simulink model "NetworkModelIntermediateIntersectionSimpleDroneModel"  (R2018b)
settings: Solver=VariableStepAuto  StartTime=tStart  StopTime=tFinal  FixedStep=0.001  RelTol=1e-3
values from neighbouring files (symbols this model uses):
  bx = 50    [MotionModelling.m]
  by = 50    [MotionModelling.m]
  ConflictDrone1andDrone2 = ControlDetectionFunction(tout,PositionXDrone1TEST, PositionYDrone1TEST, PositionXDrone2TEST, PositionYDrone2TEST, ConflictDrone1andDrone2)    [ConflictDetectionTEST.m]
  ConflictDrone1andDrone3 = ControlDetectionFunction(tout,PositionXDrone1TEST, PositionYDrone1TEST, PositionXDrone3TEST, PositionYDrone3TEST, ConflictDrone1andDrone3)    [ConflictDetectionTEST.m]
  ConflictDrone1andDrone4 = ControlDetectionFunction(tout,PositionXDrone1TEST, PositionYDrone1TEST, PositionXDrone4TEST, PositionYDrone4TEST, ConflictDrone1andDrone4)    [ConflictDetectionTEST.m]
  ConflictDrone1andDrone5 = ControlDetectionFunction(tout,PositionXDrone1TEST, PositionYDrone1TEST, PositionXDrone5TEST, PositionYDrone5TEST, ConflictDrone1andDrone5)    [ConflictDetectionTEST.m]
  ConflictDrone1andDrone6 = ControlDetectionFunction(tout,PositionXDrone1TEST, PositionYDrone1TEST, PositionXDrone6TEST, PositionYDrone6TEST, ConflictDrone1andDrone6)    [ConflictDetectionTEST.m]
  ConflictDrone1andDrone7 = ControlDetectionFunction(tout,PositionXDrone1TEST, PositionYDrone1TEST, PositionXDrone7TEST, PositionYDrone7TEST, ConflictDrone1andDrone7)    [ConflictDetectionTEST.m]
  ConflictDrone2andDrone3 = ControlDetectionFunction(tout,PositionXDrone2TEST, PositionYDrone2TEST, PositionXDrone3TEST, PositionYDrone3TEST, ConflictDrone2andDrone3)    [ConflictDetectionTEST.m]
  ConflictDrone2andDrone4 = ControlDetectionFunction(tout,PositionXDrone2, PositionYDrone2, PositionXDrone4, PositionYDrone4, ConflictDrone2andDrone4)    [ConflictDetection.m]    (also in ConflictDetectionTEST.m = ControlDetectionFunction(tout,PositionXDrone2TEST, PositionY)
  ConflictDrone2andDrone5 = ControlDetectionFunction(tout,PositionXDrone2TEST, PositionYDrone2TEST, PositionXDrone5TEST, PositionYDrone5TEST, ConflictDrone2andDrone5)    [ConflictDetectionTEST.m]
  ConflictDrone2andDrone7 = ControlDetectionFunction(tout,PositionXDrone2TEST, PositionYDrone2TEST, PositionXDrone7TEST, PositionYDrone7TEST, ConflictDrone2andDrone7)    [ConflictDetectionTEST.m]
  ConflictDrone2andDrone8 = ControlDetectionFunction(tout,PositionXDrone2TEST, PositionYDrone2TEST, PositionXDrone8TEST, PositionYDrone8TEST, ConflictDrone2andDrone8)    [ConflictDetectionTEST.m]
  ConflictDrone3andDrone4 = ControlDetectionFunction(tout,PositionXDrone3TEST, PositionYDrone3TEST, PositionXDrone4TEST, PositionYDrone4TEST, ConflictDrone3andDrone4)    [ConflictDetectionTEST.m]
  ConflictDrone3andDrone5 = ControlDetectionFunction(tout,PositionXDrone3TEST, PositionYDrone3TEST, PositionXDrone5TEST, PositionYDrone5TEST, ConflictDrone3andDrone5)    [ConflictDetectionTEST.m]
  ConflictDrone3andDrone6 = ControlDetectionFunction(tout,PositionXDrone3TEST, PositionYDrone3TEST, PositionXDrone6TEST, PositionYDrone6TEST, ConflictDrone3andDrone6)    [ConflictDetectionTEST.m]
  ConflictDrone3andDrone7 = ControlDetectionFunction(tout,PositionXDrone3TEST, PositionYDrone3TEST, PositionXDrone7TEST, PositionYDrone7TEST, ConflictDrone3andDrone7)    [ConflictDetectionTEST.m]
  ConflictDrone4andDrone6 = ControlDetectionFunction(tout,PositionXDrone4TEST, PositionYDrone4TEST, PositionXDrone6TEST, PositionYDrone6TEST, ConflictDrone4andDrone6)    [ConflictDetectionTEST.m]
  ConflictDrone5andDrone7 = ControlDetectionFunction(tout,PositionXDrone5TEST, PositionYDrone5TEST, PositionXDrone7TEST, PositionYDrone7TEST, ConflictDrone5andDrone7)    [ConflictDetectionTEST.m]
  ConflictDrone5andDrone8 = ControlDetectionFunction(tout,PositionXDrone5TEST, PositionYDrone5TEST, PositionXDrone8TEST, PositionYDrone8TEST, ConflictDrone5andDrone8)    [ConflictDetectionTEST.m]
  ConflictDrone7andDrone8 = ControlDetectionFunction(tout,PositionXDrone7TEST, PositionYDrone7TEST, PositionXDrone8TEST, PositionYDrone8TEST, ConflictDrone7andDrone8)    [ConflictDetectionTEST.m]
  deltaVx1 = 0.1*cosd (theta2)    [MotionModelling.m]
  deltaVx2 = 0.12*cosd (theta2)    [MotionModelling.m]
  deltaVx3 = 0    [MotionModelling.m]
  deltaVx4 = -0.01*cosd (theta4)    [MotionModelling.m]
  deltaVx5 = 0.02*cosd (theta5)    [MotionModelling.m]
  deltaVx7 = 0    [MotionModelling.m]
  deltaVy1 = 0    [MotionModelling.m]
  deltaVy2 = 0.12*sind (theta2)    [MotionModelling.m]
  deltaVy3 = 0.03*sind (theta3)    [MotionModelling.m]
  deltaVy4 = -0.01*sind (theta4)    [MotionModelling.m]
  deltaVy5 = 0    [MotionModelling.m]
  deltaVy6 = -0.13*sind (theta6)    [MotionModelling.m]
  deltaVy7 = -0.04*sind (theta7)    [MotionModelling.m]
  m = 1.68    [DroneSubsystemModelling.m]    (also in MotionModelling.m = 1.38)
  VelocityStarX1 = vx10    [MotionModelling.m]
  VelocityStarX2 = vx20    [MotionModelling.m]
  VelocityStarX3 = vx30    [MotionModelling.m]
  VelocityStarX4 = vx40    [MotionModelling.m]
  VelocityStarX5 = vx50    [MotionModelling.m]
  VelocityStarX6 = vx60    [MotionModelling.m]
  VelocityStarX7 = vx70    [MotionModelling.m]
  VelocityStarX8 = vx80    [MotionModelling.m]
  VelocityStarY1 = vy10    [MotionModelling.m]
  VelocityStarY2 = vy20    [MotionModelling.m]
  VelocityStarY3 = vy30    [MotionModelling.m]
  VelocityStarY4 = vy40    [MotionModelling.m]
  VelocityStarY5 = vy50    [MotionModelling.m]
  VelocityStarY6 = vy60    [MotionModelling.m]
  VelocityStarY7 = vy70    [MotionModelling.m]
  VelocityStarY8 = vy80    [MotionModelling.m]
  vx10 = vin1*cosd (theta1)    [MotionModelling.m]
  vx20 = vin2*cosd (theta2)    [MotionModelling.m]
  vx30 = vin3*cosd (theta3)    [MotionModelling.m]
  vx40 = vin4*cosd (theta4)    [MotionModelling.m]
  vx50 = vin5*cosd (theta5)    [MotionModelling.m]
  vx60 = vin6*cosd (theta6)    [MotionModelling.m]
  vx70 = vin7*cosd (theta7)    [MotionModelling.m]
  vx80 = vin2*cosd (theta8)    [MotionModelling.m]
  vy10 = vin1*sind (theta1)    [MotionModelling.m]
  vy20 = vin2*sind (theta2)    [MotionModelling.m]
  vy30 = vin3*sind (theta3)    [MotionModelling.m]
  vy40 = vin4*sind (theta4)    [MotionModelling.m]
  vy50 = vin5*sind (theta5)    [MotionModelling.m]
  vy60 = vin6*sind (theta6)    [MotionModelling.m]
  vy70 = vin7*sind (theta7)    [MotionModelling.m]
  vy80 = vin2*sind (theta8)    [MotionModelling.m]
  x10 = 10    [MotionModelling.m]
  x20 = 10    [MotionModelling.m]
  x30 = 0    [MotionModelling.m]
  x40 = -10    [MotionModelling.m]
  x50 = -10    [MotionModelling.m]
  x60 = -10    [MotionModelling.m]
  x70 = 0    [MotionModelling.m]
  x80 = 10    [MotionModelling.m]
  y10 = 0    [MotionModelling.m]
  y20 = 10    [MotionModelling.m]
  y30 = 10    [MotionModelling.m]
  y40 = 10    [MotionModelling.m]
  y50 = 0    [MotionModelling.m]
  y60 = -10    [MotionModelling.m]
  y70 = -10    [MotionModelling.m]
  y80 = -10    [MotionModelling.m]
libraries: simulink x16
settings Model: Creator=CowUser  LastModifiedBy=n9544798

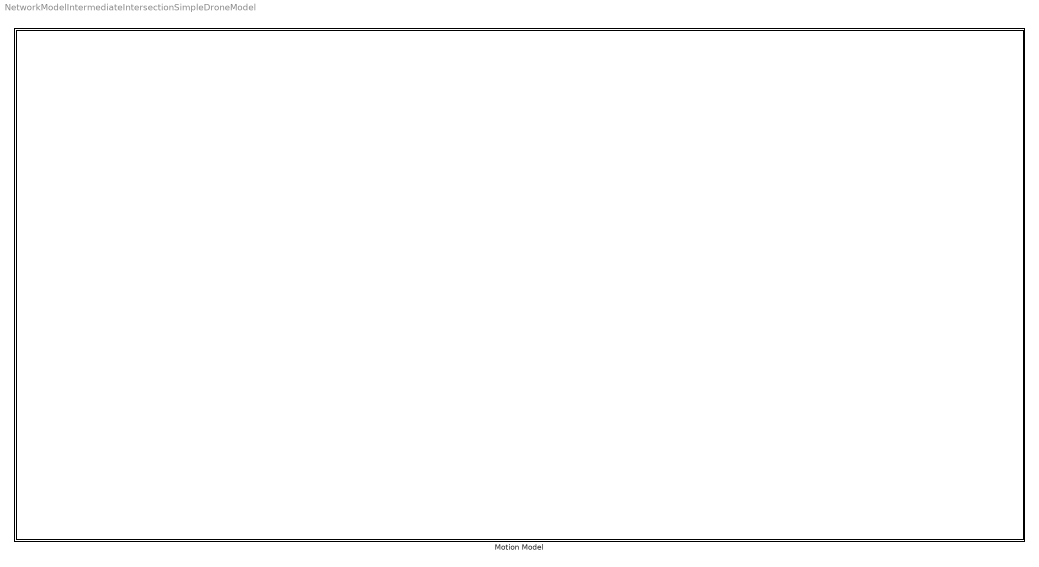
== system NetworkModelIntermediateIntersectionSimpleDroneModel ==
  Motion Model : Subsystem

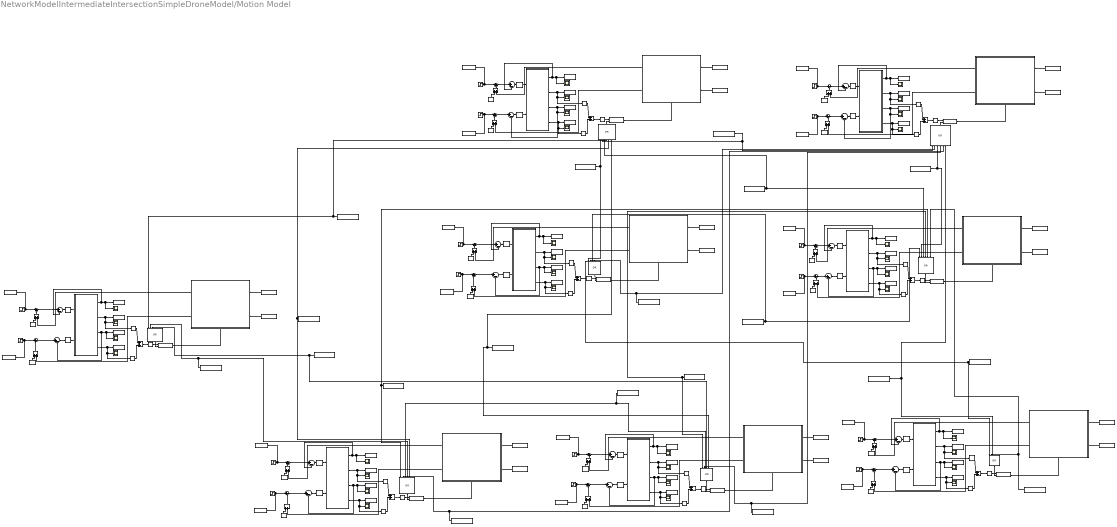
== system NetworkModelIntermediateIntersectionSimpleDroneModel/Motion Model ==
  note: Drone 2
  note: Intermediate Intersection
  note: Drone 4
  note: Sample 1
  note: Drone 1
  note: Drone 3
  note: Sample 2
  note: Sample 3
  note: Sample 4
  note: Sample 5
  note: Sample 6
  note: Sample 7
  note: Drone 5
  note: Sample 8
  note: Drone 7
  note: Sample 10
  note: Sample 9
  note: Sample 11
  note: Sample 13
  note: Sample 12
  note: Drone 6
  note: Sample 14
  note: Drone 4
  note: Sample 19
  note: Sample 18
  note: Sample 17
  note: Sample 16
  note: Sample 15
  Add{,1..23} (24 alike) : Sum
  Constant : Constant  Value=deltaVy2
  Constant1 : Constant  Value=ConflictDrone2andDrone4
  Constant10 : Constant  Value=ConflictDrone1andDrone3
  Constant11 : Constant  Value=deltaVy3
  Constant12 : Constant  Value=deltaVx1
  Constant{4..5,7..8,13..14,16..17,25..26,31..32,38..39,45..46} (16 alike) : Constant  Value=0
  Constant15 : Constant  Value=deltaVx3
  Constant18 : Constant  Value=ConflictDrone1andDrone4
  Constant19 : Constant  Value=ConflictDrone1andDrone2
  Constant2 : Constant  Value=deltaVy4
  Constant20 : Constant  Value=ConflictDrone3andDrone4
  Constant21 : Constant  Value=ConflictDrone2andDrone3
  Constant22 : Constant  Value=ConflictDrone1andDrone5
  Constant23 : Constant  Value=deltaVy5
  Constant24 : Constant  Value=deltaVx5
  Constant27 : Constant  Value=ConflictDrone3andDrone5
  Constant28 : Constant  Value=ConflictDrone1andDrone7
  Constant29 : Constant  Value=deltaVy7
  Constant3 : Constant  Value=deltaVx2
  Constant30 : Constant  Value=deltaVx7
  Constant33 : Constant  Value=ConflictDrone3andDrone7
  Constant34 : Constant  Value=ConflictDrone5andDrone7
  Constant35 : Constant  Value=ConflictDrone3andDrone6
  Constant36 : Constant  Value=deltaVy6
  Constant37 : Constant  Value=deltaVx5
  Constant40 : Constant  Value=ConflictDrone4andDrone6
  Constant41 : Constant  Value=ConflictDrone1andDrone6
  Constant42 : Constant  Value=ConflictDrone7andDrone8
  Constant43 : Constant  Value=deltaVy4
  Constant44 : Constant  Value=deltaVx4
  Constant47 : Constant  Value=ConflictDrone5andDrone8
  Constant48 : Constant  Value=ConflictDrone2andDrone8
  Constant49 : Constant  Value=ConflictDrone2andDrone7
  Constant50 : Constant  Value=ConflictDrone2andDrone5
  Constant6 : Constant  Value=deltaVx4
  Constant9 : Constant  Value=deltaVy1
  "Drone1 Subsystem " : Subsystem
  "Drone2 Subsystem " : Subsystem
  Drone3 Subsystem : Subsystem
  "Drone4 Subsystem " : Subsystem
  Drone5 Subsystem : Subsystem
  Drone6 Subsystem : Subsystem
  Drone7 Subsystem : Subsystem
  "Drone8 Subsystem " : Subsystem
  If Action Subsystem : Subsystem  TreatAsAtomicUnit=on
  If Action Subsystem1 : Subsystem  TreatAsAtomicUnit=on
  If Action Subsystem2 : Subsystem  TreatAsAtomicUnit=on
  If Action Subsystem3 : Subsystem  TreatAsAtomicUnit=on
  If Action Subsystem4 : Subsystem  TreatAsAtomicUnit=on
  If Action Subsystem5 : Subsystem  TreatAsAtomicUnit=on
  If Action Subsystem6 : Subsystem  TreatAsAtomicUnit=on
  If Action Subsystem7 : Subsystem  TreatAsAtomicUnit=on
  If{1..8} (8 alike) : If  NumInputs=2  IfExpression=(u1 <= R)&(u2 == 1)  ShowElse=off
  OR{,1..7} (8 alike) : Logic  Operator=OR  Inputs=7  IconShape=distinctive  AllPortsSameDT=off  OutDataTypeStr='double'
  PID Controller{1..16} (16 alike) : simulink/Continuous/PID Controller  Controller=PID  Form=Parallel  TimeDomain=Continuous-time  SampleTime=-1  IntegratorMethod=Forward Euler  FilterMethod=Forward Euler  ControllerParametersSource=internal  P=1.97139727738968e-05  I=1.5233344900537e-08  D=0.00566857635684116  UseFilter=on  N=15.1370363747334  TunerSelectOption=Transfer Function Based (PID Tuner App)  InitialConditionSource=internal  InitialConditionForIntegrator=0  InitialConditionForFilter=0  DifferentiatorICPrevScaledInput=0  ExternalReset=none  TrackingMode=off  Kt=1  LimitOutput=off  UpperSaturationLimit=inf  LowerSaturationLimit=-inf  LinearizeAsGain=on  AntiWindupMode=none  Kb=1  POutMin=[]  POutMax=[]  IOutMin=[]  IOutMax=[]  DOutMin=[]  DOutMax=[]  NOutMin=[]  NOutMax=[]  SumOutMin=[]  SumOutMax=[]  SaturationOutMin=[]  SaturationOutMax=[]  PParamMin=[]  PParamMax=[]  IParamMin=[]  IParamMax=[]  DParamMin=[]  DParamMax=[]  NParamMin=[]  NParamMax=[]  KbParamMin=[]  KbParamMax=[]  KtParamMin=[]  KtParamMax=[]  KbOutMin=[]  KbOutMax=[]  KtOutMin=[]  KtOutMax=[]  IntegratorOutMin=[]  IntegratorOutMax=[]  FilterOutMin=[]  FilterOutMax=[]  SumI1OutMin=[]  SumI1OutMax=[]  SumI2OutMin=[]  SumI2OutMax=[]  SumI3OutMin=[]  SumI3OutMax=[]  SumI4OutMin=[]  SumI4OutMax=[]  SumDOutMin=[]  SumDOutMax=[]  DifferentiatorOutMin=[]  DifferentiatorOutMax=[]  FilterDiffOutCoefMin=[]  FilterDiffOutCoefMax=[]  ReciprocalOutMin=[]  ReciprocalOutMax=[]  SumDenOutMin=[]  SumDenOutMax=[]  SumNumOutMin=[]  SumNumOutMax=[]  DivideOutMin=[]  DivideOutMax=[]  IntegratorContinuousStateAttributes=''  IntegratorStateMustResolveToSignalObject=off  IntegratorRTWStateStorageClass=Auto  FilterContinuousStateAttributes=''  FilterStateMustResolveToSignalObject=off  FilterRTWStateStorageClass=Auto  ParallelPVariant=InternalParameters  IdealPVariant=Disabled  IVariant=InternalParameters  DVariant=InternalParameters  IntegratorVariant=Continuous  SatVariant=Disabled  AWVariant=Passthrough  PCopyVariant=Disabled  TRVariant=Disabled  FdbkBlocksVariant=Forward  IdealPFdbkVariant=Disabled  SatFdbkVariant=Disabled  DerivativeFilterVariant=ContFilter  NVariant=InternalParameters  NCopyVariant=Disabled  FilterICVariant=InternalICsFilter  IntegratorICVariant=InternalICs  ExternalResetVariant=Disabled  TRSumVariant=Passthrough  SumFdbkVariant=Disabled  SumVariant=Sum_PID
  PositionXDrone{1..8} (8 alike) : Scope
  PositionYDrone{1..8} (8 alike) : Scope
  Sqrt{,1..7} (8 alike) : Sqrt  SaturateOnIntegerOverflow=on
  Square{,1..15} (16 alike) : Math  Operator=square  SaturateOnIntegerOverflow=on
  Step 1 : Step  Time=0  After=VelocityStarX2  SampleTime=0
  Step 10 : Step  Time=0  After=VelocityStarY5  SampleTime=0
  Step 11 : Step  Time=0  After=VelocityStarY7  SampleTime=0
  Step 12 : Step  Time=0  After=VelocityStarX7  SampleTime=0
  Step 13 : Step  Time=0  After=VelocityStarY6  SampleTime=0
  Step 14 : Step  Time=0  After=VelocityStarX6  SampleTime=0
  Step 15 : Step  Time=0  After=VelocityStarX8  SampleTime=0
  Step 16 : Step  Time=0  After=VelocityStarY8  SampleTime=0
  Step 2 : Step  Time=0  After=VelocityStarY2  SampleTime=0
  Step 3 : Step  Time=0  After=VelocityStarX1  SampleTime=0
  Step 4 : Step  Time=0  After=VelocityStarY1  SampleTime=0
  Step 5 : Step  Time=0  After=VelocityStarX3  SampleTime=0
  Step 6 : Step  Time=0  After=VelocityStarY3  SampleTime=0
  Step 7 : Step  Time=0  After=VelocityStarX4  SampleTime=0
  Step 8 : Step  Time=0  After=VelocityStarY4  SampleTime=0
  Step 9 : Step  Time=0  After=VelocityStarX5  SampleTime=0
  Sum{1..32} (32 alike) : Sum  Inputs=|+-
  To Workspace1 : ToWorkspace  VariableName=VelocityStarY2  SampleTime=-1
  To Workspace10 : ToWorkspace  VariableName=VelocityYDrone3  SampleTime=-1
  To Workspace11 : ToWorkspace  VariableName=PositionXDrone3  SampleTime=-1
  To Workspace12 : ToWorkspace  VariableName=VelocityXDrone3  SampleTime=-1
  To Workspace13 : ToWorkspace  VariableName=VelocityStarX3  SampleTime=-1
  To Workspace14 : ToWorkspace  VariableName=PositionYDrone3  SampleTime=-1
  To Workspace15 : ToWorkspace  VariableName=PositionXDrone1  SampleTime=-1
  To Workspace16 : ToWorkspace  VariableName=VelocityXDrone1  SampleTime=-1
  To Workspace17 : ToWorkspace  VariableName=VelocityStarX1  SampleTime=-1
  To Workspace18 : ToWorkspace  VariableName=PositionYDrone1  SampleTime=-1
  To Workspace19 : ToWorkspace  VariableName=VelocityStarY4  SampleTime=-1
  To Workspace2 : ToWorkspace  VariableName=VelocityYDrone2  SampleTime=-1
  To Workspace20 : ToWorkspace  VariableName=VelocityYDrone4  SampleTime=-1
  To Workspace21 : ToWorkspace  VariableName=PositionXDrone4  SampleTime=-1
  To Workspace22 : ToWorkspace  VariableName=VelocityXDrone4  SampleTime=-1
  To Workspace23 : ToWorkspace  VariableName=VelocityStarX4  SampleTime=-1
  To Workspace24 : ToWorkspace  VariableName=PositionYDrone4  SampleTime=-1
  To Workspace25 : ToWorkspace  VariableName=VelocityStarY5  SampleTime=-1
  To Workspace26 : ToWorkspace  VariableName=VelocityYDrone5  SampleTime=-1
  To Workspace27 : ToWorkspace  VariableName=PositionXDrone5  SampleTime=-1
  To Workspace28 : ToWorkspace  VariableName=VelocityXDrone5  SampleTime=-1
  To Workspace29 : ToWorkspace  VariableName=VelocityStarX5  SampleTime=-1
  To Workspace3 : ToWorkspace  VariableName=PositionXDrone2  SampleTime=-1
  To Workspace30 : ToWorkspace  VariableName=PositionYDrone5  SampleTime=-1
  To Workspace31 : ToWorkspace  VariableName=VelocityStarY7  SampleTime=-1
  To Workspace32 : ToWorkspace  VariableName=VelocityYDrone7  SampleTime=-1
  To Workspace33 : ToWorkspace  VariableName=PositionXDrone7  SampleTime=-1
  To Workspace34 : ToWorkspace  VariableName=VelocityXDrone7  SampleTime=-1
  To Workspace35 : ToWorkspace  VariableName=VelocityStarX7  SampleTime=-1
  To Workspace36 : ToWorkspace  VariableName=PositionYDrone7  SampleTime=-1
  To Workspace37 : ToWorkspace  VariableName=VelocityStarY6  SampleTime=-1
  To Workspace38 : ToWorkspace  VariableName=VelocityYDrone6  SampleTime=-1
  To Workspace39 : ToWorkspace  VariableName=PositionXDrone6  SampleTime=-1
  To Workspace4 : ToWorkspace  VariableName=VelocityXDrone2  SampleTime=-1
  To Workspace40 : ToWorkspace  VariableName=VelocityXDrone6  SampleTime=-1
  To Workspace41 : ToWorkspace  VariableName=VelocityStarX6  SampleTime=-1
  To Workspace42 : ToWorkspace  VariableName=PositionYDrone6  SampleTime=-1
  To Workspace43 : ToWorkspace  VariableName=VelocityStarY8  SampleTime=-1
  To Workspace44 : ToWorkspace  VariableName=VelocityYDrone8  SampleTime=-1
  To Workspace45 : ToWorkspace  VariableName=PositionXDrone8  SampleTime=-1
  To Workspace46 : ToWorkspace  VariableName=VelocityXDrone8  SampleTime=-1
  To Workspace47 : ToWorkspace  VariableName=VelocityStarX8  SampleTime=-1
  To Workspace48 : ToWorkspace  VariableName=PositionYDrone8  SampleTime=-1
  To Workspace5 : ToWorkspace  VariableName=VelocityStarX2  SampleTime=-1
  To Workspace6 : ToWorkspace  VariableName=PositionYDrone2  SampleTime=-1
  To Workspace7 : ToWorkspace  VariableName=VelocityStarY1  SampleTime=-1
  To Workspace8 : ToWorkspace  VariableName=VelocityStarY3  SampleTime=-1
  To Workspace9 : ToWorkspace  VariableName=VelocityYDrone1  SampleTime=-1
  VelocityXDrone{1..8} (8 alike) : Scope
  VelocityYDrone{1..8} (8 alike) : Scope
  wires:
  "Drone2 Subsystem "/3(VelocityY) -> Sum1/2, VelocityYDrone2/1, To Workspace2/1
  Sum1/1 -> PID Controller1/1
  PID Controller7/1 -> "Drone2 Subsystem "/1(InputForceX)
  "Drone2 Subsystem "/4(PositionY) -> Square1/1, PositionYDrone2/1, To Workspace6/1
  "Drone2 Subsystem "/2(PositionX) -> Square/1, PositionXDrone2/1, To Workspace3/1
  PID Controller1/1 -> "Drone2 Subsystem "/2(InputForceY)
  "Drone2 Subsystem "/1(VelocityX) -> VelocityXDrone2/1, To Workspace4/1, Sum2/2
  Step 7/1 -> Sum6/1, To Workspace23/1
  Step 8/1 -> To Workspace19/1, Sum7/1
  Square/1 -> Add/1
  Square1/1 -> Add/2
  Add/1 -> Sqrt/1
  Sqrt/1 -> If3/1
  Square2/1 -> Add1/1
  Add1/1 -> Sqrt1/1
  "Drone4 Subsystem "/2(PositionX) -> Square2/1, PositionXDrone4/1, To Workspace21/1
  Square3/1 -> Add1/2
  "Drone4 Subsystem "/4(PositionY) -> Square3/1, PositionYDrone4/1, To Workspace24/1
  Sqrt1/1 -> If1/1
  Sum2/1 -> PID Controller7/1
  Constant/1 -> If Action Subsystem/2(deltaVy2)
  Constant3/1 -> If Action Subsystem/1(deltaVx2)
  Step 1/1 -> Sum9/1, To Workspace5/1
  Sum10/1 -> Sum1/1
  Step 2/1 -> Sum10/1, To Workspace1/1
  If Action Subsystem/1(dVx2) -> Add3/2
  If Action Subsystem/2(dVy2) -> Add2/2
  If3/1 -> If Action Subsystem/Action
  Constant4/1 -> Add3/1
  Constant5/1 -> Add2/1
  Add2/1 -> Sum10/2
  Constant1/1 -> OR1/1, OR2/1
  If1/1 -> If Action Subsystem1/Action
  If Action Subsystem1/1(dVx4) -> Add4/2
  Constant2/1 -> If Action Subsystem1/2(deltaVy4)
  Constant6/1 -> If Action Subsystem1/1(deltaVx4)
  Add4/1 -> Sum6/2
  Constant7/1 -> Add4/1
  Sum3/1 -> PID Controller6/1
  "Drone4 Subsystem "/1(VelocityX) -> Sum3/2, To Workspace22/1, VelocityXDrone4/1
  Constant8/1 -> Add5/1
  If Action Subsystem1/2(dVy4) -> Add5/2
  "Drone4 Subsystem "/3(VelocityY) -> Sum4/2, VelocityYDrone4/1, To Workspace20/1
  Sum4/1 -> PID Controller3/1
  Add3/1 -> Sum9/2
  Sum9/1 -> Sum2/1
  Step 3/1 -> Sum16/1, To Workspace17/1
  Add9/1 -> Sum16/2
  "Drone1 Subsystem "/4(PositionY) -> Square5/1, PositionYDrone1/1, To Workspace18/1
  Drone3 Subsystem/3(VelocityY) -> Sum13/2, VelocityYDrone3/1, To Workspace10/1
  Constant17/1 -> Add11/1
  Add10/1 -> Sum14/2
  Sum15/1 -> Sum13/1
  If Action Subsystem3/2(dVy3) -> Add11/2
  Add11/1 -> Sum15/2
  Sum11/1 -> PID Controller8/1
  Constant10/1 -> OR3/2, OR/3
  If Action Subsystem2/1(dVx1) -> Add9/2
  Constant11/1 -> If Action Subsystem3/2(deltaVy3)
  Constant13/1 -> Add9/1
  Sqrt3/1 -> If2/1
  Constant16/1 -> Add10/1
  Add8/1 -> Sum8/2
  Drone3 Subsystem/1(VelocityX) -> Sum12/2, To Workspace12/1, VelocityXDrone3/1
  Constant14/1 -> Add8/1
  If2/1 -> If Action Subsystem3/Action
  If Action Subsystem3/1(dVx3) -> Add10/2
  Drone3 Subsystem/4(PositionY) -> Square7/1, PositionYDrone3/1, To Workspace14/1
  Constant12/1 -> If Action Subsystem2/1(deltaVx1)
  Constant15/1 -> If Action Subsystem3/1(deltaVx3)
  Step 4/1 -> Sum8/1, To Workspace7/1
  "Drone1 Subsystem "/2(PositionX) -> Square4/1, PositionXDrone1/1, To Workspace15/1
  Add7/1 -> Sqrt3/1
  Square6/1 -> Add7/1
  Square5/1 -> Add6/2
  Constant9/1 -> If Action Subsystem2/2(deltaVy1)
  Square7/1 -> Add7/2
  Sum13/1 -> PID Controller5/1
  Drone3 Subsystem/2(PositionX) -> Square6/1, PositionXDrone3/1, To Workspace11/1
  Sum14/1 -> Sum12/1
  Step 5/1 -> Sum14/1, To Workspace13/1
  Sum12/1 -> PID Controller4/1
  Step 6/1 -> To Workspace8/1, Sum15/1
  Sum5/1 -> PID Controller2/1
  Sqrt2/1 -> If4/1
  PID Controller4/1 -> Drone3 Subsystem/1(InputForceX)
  Add6/1 -> Sqrt2/1
  PID Controller5/1 -> Drone3 Subsystem/2(InputForceY)
  "Drone1 Subsystem "/3(VelocityY) -> Sum5/2, VelocityYDrone1/1, To Workspace9/1
  If Action Subsystem2/2(dVy1) -> Add8/2
  Square4/1 -> Add6/1
  If4/1 -> If Action Subsystem2/Action
  "Drone1 Subsystem "/1(VelocityX) -> VelocityXDrone1/1, To Workspace16/1, Sum11/2
  OR/1 -> If4/2
  Constant18/1 -> OR/2, OR1/2
  OR1/1 -> If1/2
  OR2/1 -> If3/2
  Constant19/1 -> OR2/2, OR/1
  Constant20/1 -> OR3/1, OR1/3
  OR3/1 -> If2/2
  Constant21/1 -> OR3/3, OR2/3
  Sum6/1 -> Sum3/1
  Sum8/1 -> Sum5/1
  Sum16/1 -> Sum11/1
  Add5/1 -> Sum7/2
  Sum7/1 -> Sum4/1
  PID Controller6/1 -> "Drone4 Subsystem "/1(InputForceX)
  PID Controller3/1 -> "Drone4 Subsystem "/2(InputForceY)
  Constant26/1 -> Add14/1
  Constant25/1 -> Add13/1
  Sum17/1 -> PID Controller10/1
  Drone5 Subsystem/1(VelocityX) -> Sum17/2, To Workspace28/1, VelocityXDrone5/1
  Drone5 Subsystem/2(PositionX) -> Square8/1, PositionXDrone5/1, To Workspace27/1
  Step 10/1 -> To Workspace25/1, Sum20/1
  Square8/1 -> Add12/1
  PID Controller10/1 -> Drone5 Subsystem/1(InputForceX)
  Drone5 Subsystem/3(VelocityY) -> Sum18/2, VelocityYDrone5/1, To Workspace26/1
  Sum20/1 -> Sum18/1
  Sqrt4/1 -> If5/1
  If5/1 -> If Action Subsystem4/Action
  Sum18/1 -> PID Controller9/1
  PID Controller9/1 -> Drone5 Subsystem/2(InputForceY)
  Sum19/1 -> Sum17/1
  If Action Subsystem4/1(dVx5) -> Add13/2
  Add14/1 -> Sum20/2
  Constant23/1 -> If Action Subsystem4/2(deltaVy5)
  Constant22/1 -> OR/4, OR4/2
  Step 9/1 -> Sum19/1, To Workspace29/1
  If Action Subsystem4/2(dVy5) -> Add14/2
  Square9/1 -> Add12/2
  Constant24/1 -> If Action Subsystem4/1(deltaVx5)
  Drone5 Subsystem/4(PositionY) -> Square9/1, PositionYDrone5/1, To Workspace30/1
  Add13/1 -> Sum19/2
  OR4/1 -> If5/2
  Add12/1 -> Sqrt4/1
  Constant27/1 -> OR3/4, OR4/1
  OR5/1 -> If6/2
  Constant30/1 -> If Action Subsystem5/1(deltaVx7)
  Drone7 Subsystem/4(PositionY) -> Square11/1, PositionYDrone7/1, To Workspace36/1
  If Action Subsystem5/2(dVy7) -> Add17/2
  Add16/1 -> Sum23/2
  Add15/1 -> Sqrt5/1
  Constant28/1 -> OR/5, OR5/2
  Constant29/1 -> If Action Subsystem5/2(deltaVy7)
  Square11/1 -> Add15/2
  Add17/1 -> Sum24/2
  If Action Subsystem5/1(dVx7) -> Add16/2
  Constant34/1 -> OR4/3, OR5/3
  Constant33/1 -> OR3/5, OR5/1
  Sum22/1 -> PID Controller12/1
  Sum24/1 -> Sum22/1
  If6/1 -> If Action Subsystem5/Action
  Step 12/1 -> Sum23/1, To Workspace35/1
  Drone7 Subsystem/3(VelocityY) -> Sum22/2, VelocityYDrone7/1, To Workspace32/1
  Drone7 Subsystem/2(PositionX) -> Square10/1, PositionXDrone7/1, To Workspace33/1
  PID Controller11/1 -> Drone7 Subsystem/1(InputForceX)
  Square10/1 -> Add15/1
  Step 11/1 -> To Workspace31/1, Sum24/1
  Constant31/1 -> Add16/1
  Sum21/1 -> PID Controller11/1
  Sqrt5/1 -> If6/1
  Drone7 Subsystem/1(VelocityX) -> Sum21/2, To Workspace34/1, VelocityXDrone7/1
  Sum23/1 -> Sum21/1
  Constant32/1 -> Add17/1
  Add20/1 -> Sum28/2
  Square12/1 -> Add18/1
  Sum27/1 -> Sum25/1
  PID Controller14/1 -> Drone6 Subsystem/2(InputForceY)
  Square13/1 -> Add18/2
  PID Controller13/1 -> Drone6 Subsystem/1(InputForceX)
  Drone6 Subsystem/3(VelocityY) -> Sum26/2, VelocityYDrone6/1, To Workspace38/1
  Drone6 Subsystem/4(PositionY) -> Square13/1, PositionYDrone6/1, To Workspace42/1
  Constant38/1 -> Add19/1
  Constant40/1 -> OR1/4, OR6/1
  OR6/1 -> If7/2
  Sum25/1 -> PID Controller13/1
  Sqrt6/1 -> If7/1
  If Action Subsystem6/2(dVy6) -> Add20/2
  Constant35/1 -> OR3/6, OR6/2
  Constant39/1 -> Add20/1
  Sum28/1 -> Sum26/1
  If Action Subsystem6/1(dVx6) -> Add19/2
  Step 13/1 -> To Workspace37/1, Sum28/1
  If7/1 -> If Action Subsystem6/Action
  Constant41/1 -> OR6/3, OR/6
  Add19/1 -> Sum27/2
  Step 14/1 -> Sum27/1, To Workspace41/1
  Sum26/1 -> PID Controller14/1
  Drone6 Subsystem/2(PositionX) -> Square12/1, PositionXDrone6/1, To Workspace39/1
  Add18/1 -> Sqrt6/1
  Constant36/1 -> If Action Subsystem6/2(deltaVy6)
  Constant37/1 -> If Action Subsystem6/1(deltaVx6)
  Drone6 Subsystem/1(VelocityX) -> Sum25/2, To Workspace40/1, VelocityXDrone6/1
  Step 16/1 -> To Workspace43/1, Sum32/1
  If Action Subsystem7/1(dVx4) -> Add22/2
  Constant48/1 -> OR2/4, OR7/1
  Constant43/1 -> If Action Subsystem7/2(deltaVy4)
  Add21/1 -> Sqrt7/1
  Square14/1 -> Add21/1
  Constant46/1 -> Add23/1
  If8/1 -> If Action Subsystem7/Action
  Sum30/1 -> PID Controller15/1
  "Drone8 Subsystem "/1(VelocityX) -> Sum29/2, To Workspace46/1, VelocityXDrone8/1
  Constant47/1 -> OR4/4, OR7/3
  "Drone8 Subsystem "/3(VelocityY) -> Sum30/2, VelocityYDrone8/1, To Workspace44/1
  "Drone8 Subsystem "/2(PositionX) -> Square14/1, PositionXDrone8/1, To Workspace45/1
  Sqrt7/1 -> If8/1
  Add23/1 -> Sum32/2
  OR7/1 -> If8/2
  PID Controller15/1 -> "Drone8 Subsystem "/2(InputForceY)
  If Action Subsystem7/2(dVy4) -> Add23/2
  Square15/1 -> Add21/2
  Sum32/1 -> Sum30/1
  Constant45/1 -> Add22/1
  "Drone8 Subsystem "/4(PositionY) -> Square15/1, PositionYDrone8/1, To Workspace48/1
  Constant44/1 -> If Action Subsystem7/1(deltaVx4)
  Step 15/1 -> Sum31/1, To Workspace47/1
  Sum29/1 -> PID Controller16/1
  Add22/1 -> Sum31/2
  PID Controller16/1 -> "Drone8 Subsystem "/1(InputForceX)
  Sum31/1 -> Sum29/1
  Constant42/1 -> OR5/4, OR7/2
  Constant49/1 -> OR2/5, OR5/5
  Constant50/1 -> OR2/6, OR4/5
  PID Controller8/1 -> "Drone1 Subsystem "/1(InputForceX)
  PID Controller2/1 -> "Drone1 Subsystem "/2(InputForceY)
  PID Controller12/1 -> Drone7 Subsystem/2(InputForceY)

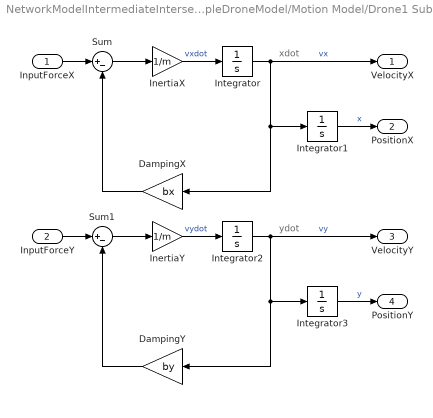
== system NetworkModelIntermediateIntersectionSimpleDroneModel/Motion Model/Drone1 Subsystem  ==
  note: ydot
  note: xdot
  InputForceX : Inport
  InputForceY : Inport  Port=2
  DampingX : Gain  Gain=bx
  DampingY : Gain  Gain=by
  InertiaX : Gain  Gain=1/m
  InertiaY : Gain  Gain=1/m
  Integrator : Integrator  InitialCondition=vx10
  Integrator1 : Integrator  InitialCondition=x10
  Integrator2 : Integrator  InitialCondition=vy10
  Integrator3 : Integrator  InitialCondition=y10
  Sum : Sum  Inputs=|+-
  Sum1 : Sum  Inputs=|+-
  VelocityX : Outport
  PositionX : Outport  Port=2
  VelocityY : Outport  Port=3
  PositionY : Outport  Port=4
  wires:
  InertiaX/1 -> Integrator/1  "vxdot"
  Integrator1/1 -> PositionX/1  "x"
  InputForceY/1 -> Sum1/1
  Integrator2/1 -> VelocityY/1, Integrator3/1, DampingY/1  "vy"
  InertiaY/1 -> Integrator2/1  "vydot"
  Integrator/1 -> VelocityX/1, Integrator1/1, DampingX/1  "vx"
  Sum1/1 -> InertiaY/1
  DampingY/1 -> Sum1/2
  Sum/1 -> InertiaX/1
  DampingX/1 -> Sum/2
  Integrator3/1 -> PositionY/1  "y"
  InputForceX/1 -> Sum/1

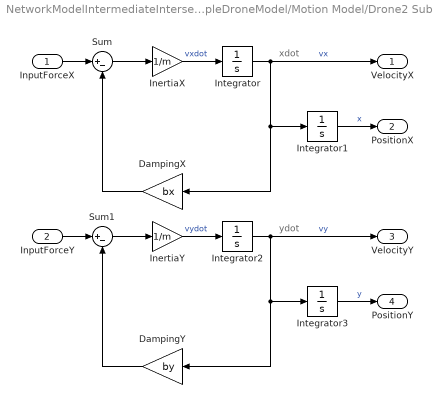
== system NetworkModelIntermediateIntersectionSimpleDroneModel/Motion Model/Drone2 Subsystem  ==
  note: ydot
  note: xdot
  InputForceX : Inport
  InputForceY : Inport  Port=2
  "DampingX " : Gain  Gain=bx
  DampingY : Gain  Gain=by
  InertiaX : Gain  Gain=1/m
  InertiaY : Gain  Gain=1/m
  Integrator : Integrator  InitialCondition=vx20
  Integrator1 : Integrator  InitialCondition=x20
  Integrator2 : Integrator  InitialCondition=vy20
  Integrator3 : Integrator  InitialCondition=y20
  Sum : Sum  Inputs=|+-
  Sum1 : Sum  Inputs=|+-
  VelocityX : Outport
  PositionX : Outport  Port=2
  VelocityY : Outport  Port=3
  PositionY : Outport  Port=4
  wires:
  InputForceY/1 -> Sum1/1
  Integrator2/1 -> VelocityY/1, Integrator3/1, DampingY/1  "vy"
  DampingY/1 -> Sum1/2
  InertiaY/1 -> Integrator2/1  "vydot"
  Integrator1/1 -> PositionX/1  "x"
  Integrator/1 -> VelocityX/1, Integrator1/1, "DampingX "/1  "vx"
  InputForceX/1 -> Sum/1
  Sum/1 -> InertiaX/1
  Integrator3/1 -> PositionY/1  "y"
  "DampingX "/1 -> Sum/2
  InertiaX/1 -> Integrator/1  "vxdot"
  Sum1/1 -> InertiaY/1

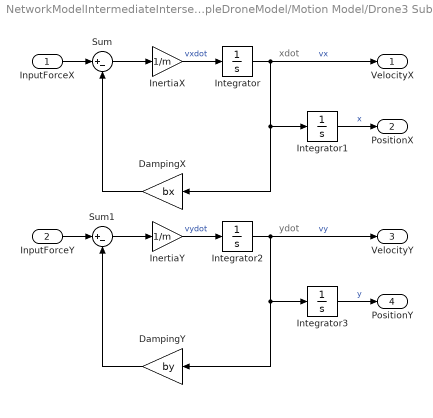
== system NetworkModelIntermediateIntersectionSimpleDroneModel/Motion Model/Drone3 Subsystem ==
  note: xdot
  note: ydot
  InputForceX : Inport
  InputForceY : Inport  Port=2
  DampingX : Gain  Gain=bx
  DampingY : Gain  Gain=by
  InertiaX : Gain  Gain=1/m
  InertiaY : Gain  Gain=1/m
  Integrator : Integrator  InitialCondition=vx30
  Integrator1 : Integrator  InitialCondition=x30
  Integrator2 : Integrator  InitialCondition=vy30
  Integrator3 : Integrator  InitialCondition=y30
  Sum : Sum  Inputs=|+-
  Sum1 : Sum  Inputs=|+-
  VelocityX : Outport
  PositionX : Outport  Port=2
  VelocityY : Outport  Port=3
  PositionY : Outport  Port=4
  wires:
  Integrator3/1 -> PositionY/1  "y"
  Integrator/1 -> VelocityX/1, Integrator1/1, DampingX/1  "vx"
  InertiaY/1 -> Integrator2/1  "vydot"
  DampingY/1 -> Sum1/2
  Sum1/1 -> InertiaY/1
  Integrator1/1 -> PositionX/1  "x"
  InputForceY/1 -> Sum1/1
  DampingX/1 -> Sum/2
  Sum/1 -> InertiaX/1
  InertiaX/1 -> Integrator/1  "vxdot"
  InputForceX/1 -> Sum/1
  Integrator2/1 -> VelocityY/1, Integrator3/1, DampingY/1  "vy"

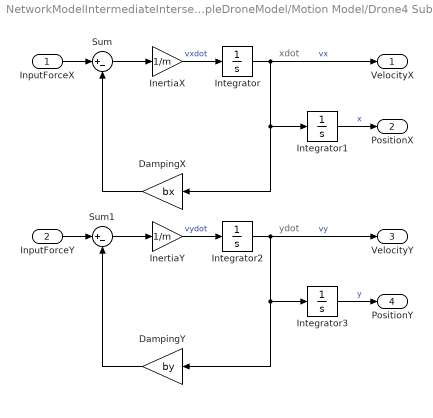
== system NetworkModelIntermediateIntersectionSimpleDroneModel/Motion Model/Drone4 Subsystem  ==
  note: xdot
  note: ydot
  InputForceX : Inport
  InputForceY : Inport  Port=2
  "DampingX " : Gain  Gain=bx
  DampingY : Gain  Gain=by
  InertiaX : Gain  Gain=1/m
  InertiaY : Gain  Gain=1/m
  Integrator : Integrator  InitialCondition=vx40
  Integrator1 : Integrator  InitialCondition=x40
  Integrator2 : Integrator  InitialCondition=vy40
  Integrator3 : Integrator  InitialCondition=y40
  Sum : Sum  Inputs=|+-
  Sum1 : Sum  Inputs=|+-
  VelocityX : Outport
  PositionX : Outport  Port=2
  VelocityY : Outport  Port=3
  PositionY : Outport  Port=4
  wires:
  Integrator1/1 -> PositionX/1  "x"
  InputForceX/1 -> Sum/1
  InertiaY/1 -> Integrator2/1  "vydot"
  InputForceY/1 -> Sum1/1
  Integrator3/1 -> PositionY/1  "y"
  Integrator2/1 -> VelocityY/1, Integrator3/1, DampingY/1  "vy"
  "DampingX "/1 -> Sum/2
  InertiaX/1 -> Integrator/1  "vxdot"
  Sum1/1 -> InertiaY/1
  Sum/1 -> InertiaX/1
  Integrator/1 -> VelocityX/1, Integrator1/1, "DampingX "/1  "vx"
  DampingY/1 -> Sum1/2

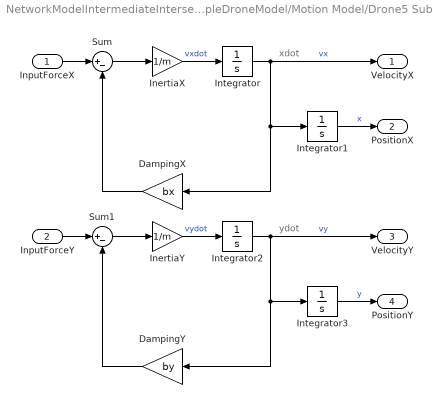
== system NetworkModelIntermediateIntersectionSimpleDroneModel/Motion Model/Drone5 Subsystem ==
  note: xdot
  note: ydot
  InputForceX : Inport
  InputForceY : Inport  Port=2
  "DampingX " : Gain  Gain=bx
  DampingY : Gain  Gain=by
  InertiaX : Gain  Gain=1/m
  InertiaY : Gain  Gain=1/m
  Integrator : Integrator  InitialCondition=vx50
  Integrator1 : Integrator  InitialCondition=x50
  Integrator2 : Integrator  InitialCondition=vy50
  Integrator3 : Integrator  InitialCondition=y50
  Sum : Sum  Inputs=|+-
  Sum1 : Sum  Inputs=|+-
  VelocityX : Outport
  PositionX : Outport  Port=2
  VelocityY : Outport  Port=3
  PositionY : Outport  Port=4
  wires:
  Integrator/1 -> VelocityX/1, Integrator1/1, "DampingX "/1  "vx"
  Sum/1 -> InertiaX/1
  Sum1/1 -> InertiaY/1
  "DampingX "/1 -> Sum/2
  Integrator3/1 -> PositionY/1  "y"
  InertiaY/1 -> Integrator2/1  "vydot"
  Integrator1/1 -> PositionX/1  "x"
  Integrator2/1 -> VelocityY/1, Integrator3/1, DampingY/1  "vy"
  InputForceY/1 -> Sum1/1
  InputForceX/1 -> Sum/1
  InertiaX/1 -> Integrator/1  "vxdot"
  DampingY/1 -> Sum1/2

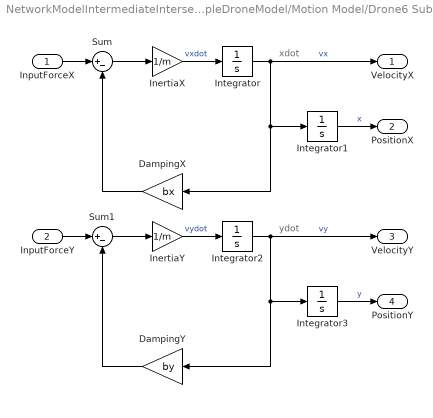
== system NetworkModelIntermediateIntersectionSimpleDroneModel/Motion Model/Drone6 Subsystem ==
  note: xdot
  note: ydot
  InputForceX : Inport
  InputForceY : Inport  Port=2
  "DampingX " : Gain  Gain=bx
  DampingY : Gain  Gain=by
  InertiaX : Gain  Gain=1/m
  InertiaY : Gain  Gain=1/m
  Integrator : Integrator  InitialCondition=vx60
  Integrator1 : Integrator  InitialCondition=x60
  Integrator2 : Integrator  InitialCondition=vy60
  Integrator3 : Integrator  InitialCondition=y60
  Sum : Sum  Inputs=|+-
  Sum1 : Sum  Inputs=|+-
  VelocityX : Outport
  PositionX : Outport  Port=2
  VelocityY : Outport  Port=3
  PositionY : Outport  Port=4
  wires:
  InputForceY/1 -> Sum1/1
  InertiaY/1 -> Integrator2/1  "vydot"
  DampingY/1 -> Sum1/2
  "DampingX "/1 -> Sum/2
  Integrator/1 -> VelocityX/1, Integrator1/1, "DampingX "/1  "vx"
  Integrator3/1 -> PositionY/1  "y"
  Sum1/1 -> InertiaY/1
  Integrator1/1 -> PositionX/1  "x"
  InputForceX/1 -> Sum/1
  Integrator2/1 -> VelocityY/1, Integrator3/1, DampingY/1  "vy"
  Sum/1 -> InertiaX/1
  InertiaX/1 -> Integrator/1  "vxdot"

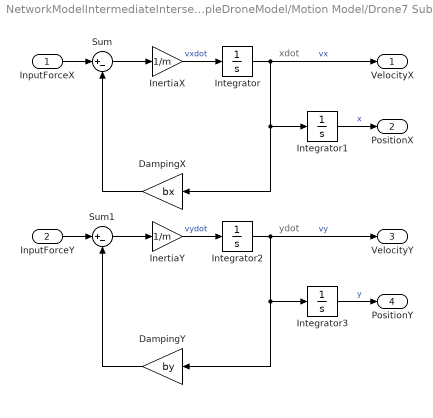
== system NetworkModelIntermediateIntersectionSimpleDroneModel/Motion Model/Drone7 Subsystem ==
  note: ydot
  note: xdot
  InputForceX : Inport
  InputForceY : Inport  Port=2
  "DampingX " : Gain  Gain=bx
  DampingY : Gain  Gain=by
  InertiaX : Gain  Gain=1/m
  InertiaY : Gain  Gain=1/m
  Integrator : Integrator  InitialCondition=vx70
  Integrator1 : Integrator  InitialCondition=x70
  Integrator2 : Integrator  InitialCondition=vy70
  Integrator3 : Integrator  InitialCondition=y70
  Sum : Sum  Inputs=|+-
  Sum1 : Sum  Inputs=|+-
  VelocityX : Outport
  PositionX : Outport  Port=2
  VelocityY : Outport  Port=3
  PositionY : Outport  Port=4
  wires:
  Integrator2/1 -> VelocityY/1, Integrator3/1, DampingY/1  "vy"
  DampingY/1 -> Sum1/2
  InertiaY/1 -> Integrator2/1  "vydot"
  Sum1/1 -> InertiaY/1
  Integrator3/1 -> PositionY/1  "y"
  InputForceX/1 -> Sum/1
  Integrator/1 -> VelocityX/1, Integrator1/1, "DampingX "/1  "vx"
  Integrator1/1 -> PositionX/1  "x"
  InputForceY/1 -> Sum1/1
  InertiaX/1 -> Integrator/1  "vxdot"
  Sum/1 -> InertiaX/1
  "DampingX "/1 -> Sum/2

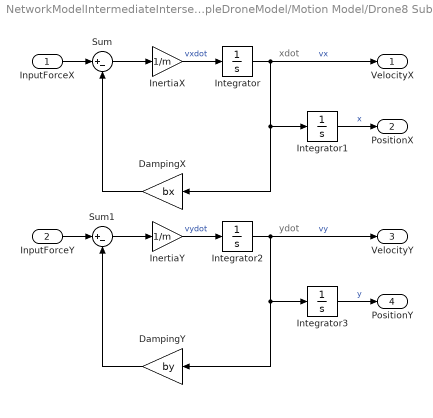
== system NetworkModelIntermediateIntersectionSimpleDroneModel/Motion Model/Drone8 Subsystem  ==
  note: xdot
  note: ydot
  InputForceX : Inport
  InputForceY : Inport  Port=2
  "DampingX " : Gain  Gain=bx
  DampingY : Gain  Gain=by
  InertiaX : Gain  Gain=1/m
  InertiaY : Gain  Gain=1/m
  Integrator : Integrator  InitialCondition=vx80
  Integrator1 : Integrator  InitialCondition=x80
  Integrator2 : Integrator  InitialCondition=vy80
  Integrator3 : Integrator  InitialCondition=y80
  Sum : Sum  Inputs=|+-
  Sum1 : Sum  Inputs=|+-
  VelocityX : Outport
  PositionX : Outport  Port=2
  VelocityY : Outport  Port=3
  PositionY : Outport  Port=4
  wires:
  Integrator2/1 -> VelocityY/1, Integrator3/1, DampingY/1  "vy"
  Integrator1/1 -> PositionX/1  "x"
  InertiaY/1 -> Integrator2/1  "vydot"
  InputForceY/1 -> Sum1/1
  "DampingX "/1 -> Sum/2
  Integrator/1 -> VelocityX/1, Integrator1/1, "DampingX "/1  "vx"
  DampingY/1 -> Sum1/2
  Sum/1 -> InertiaX/1
  InputForceX/1 -> Sum/1
  Integrator3/1 -> PositionY/1  "y"
  InertiaX/1 -> Integrator/1  "vxdot"
  Sum1/1 -> InertiaY/1

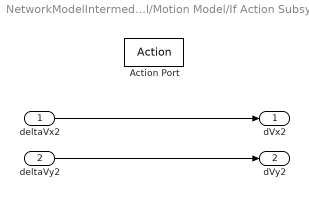
== system NetworkModelIntermediateIntersectionSimpleDroneModel/Motion Model/If Action Subsystem ==
  deltaVx2 : Inport
  deltaVy2 : Inport  Port=2
  Action Port : ActionPort  ActionType=then
  dVx2 : Outport
  dVy2 : Outport  Port=2
  wires:
  deltaVx2/1 -> dVx2/1
  deltaVy2/1 -> dVy2/1

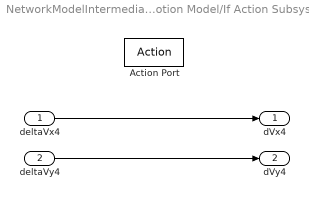
== system NetworkModelIntermediateIntersectionSimpleDroneModel/Motion Model/If Action Subsystem1 ==
  deltaVx4 : Inport
  deltaVy4 : Inport  Port=2
  Action Port : ActionPort  ActionType=then
  dVx4 : Outport
  dVy4 : Outport  Port=2
  wires:
  deltaVx4/1 -> dVx4/1
  deltaVy4/1 -> dVy4/1

== system NetworkModelIntermediateIntersectionSimpleDroneModel/Motion Model/If Action Subsystem2 ==
  deltaVx1 : Inport
  deltaVy1 : Inport  Port=2
  Action Port : ActionPort  ActionType=then
  dVx1 : Outport
  dVy1 : Outport  Port=2
  wires:
  deltaVx1/1 -> dVx1/1
  deltaVy1/1 -> dVy1/1

== system NetworkModelIntermediateIntersectionSimpleDroneModel/Motion Model/If Action Subsystem3 ==
  deltaVx3 : Inport
  deltaVy3 : Inport  Port=2
  Action Port : ActionPort  ActionType=then
  dVx3 : Outport
  dVy3 : Outport  Port=2
  wires:
  deltaVx3/1 -> dVx3/1
  deltaVy3/1 -> dVy3/1

== system NetworkModelIntermediateIntersectionSimpleDroneModel/Motion Model/If Action Subsystem4 ==
  deltaVx5 : Inport
  deltaVy5 : Inport  Port=2
  Action Port : ActionPort  ActionType=then
  dVx5 : Outport
  dVy5 : Outport  Port=2
  wires:
  deltaVx5/1 -> dVx5/1
  deltaVy5/1 -> dVy5/1

== system NetworkModelIntermediateIntersectionSimpleDroneModel/Motion Model/If Action Subsystem5 ==
  deltaVx7 : Inport
  deltaVy7 : Inport  Port=2
  Action Port : ActionPort  ActionType=then
  dVx7 : Outport
  dVy7 : Outport  Port=2
  wires:
  deltaVx7/1 -> dVx7/1
  deltaVy7/1 -> dVy7/1

== system NetworkModelIntermediateIntersectionSimpleDroneModel/Motion Model/If Action Subsystem6 ==
  deltaVx6 : Inport
  deltaVy6 : Inport  Port=2
  Action Port : ActionPort  ActionType=then
  dVx6 : Outport
  dVy6 : Outport  Port=2
  wires:
  deltaVx6/1 -> dVx6/1
  deltaVy6/1 -> dVy6/1

== system NetworkModelIntermediateIntersectionSimpleDroneModel/Motion Model/If Action Subsystem7 ==
  deltaVx4 : Inport
  deltaVy4 : Inport  Port=2
  Action Port : ActionPort  ActionType=then
  dVx4 : Outport
  dVy4 : Outport  Port=2
  wires:
  deltaVx4/1 -> dVx4/1
  deltaVy4/1 -> dVy4/1
